simulink model "vehicle_sil"  (R2022b)
settings: Solver=VariableStepAuto  StartTime=0.0  StopTime=inf  RelTol=1e-3
undefined symbols (not defined in the file or in its folder): canChannel, MI_STATUSES
libraries: canmsglib x16, canlib x10, AMK_comms_plant_lib x1, BMS_plant_lib x1, realtime_pacer_lib x1, battery_monitor_lib x1, driver_interface_lib x1, governor_lib x1, motor_interface_lib x1, simp_vd_lib x1
settings Model: Creator=LinF  LastModifiedBy=LinF

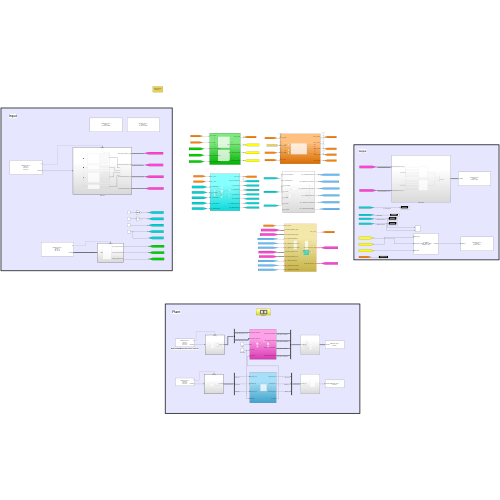
[thumbnail: Simulink's stored preview of the top-level diagram]
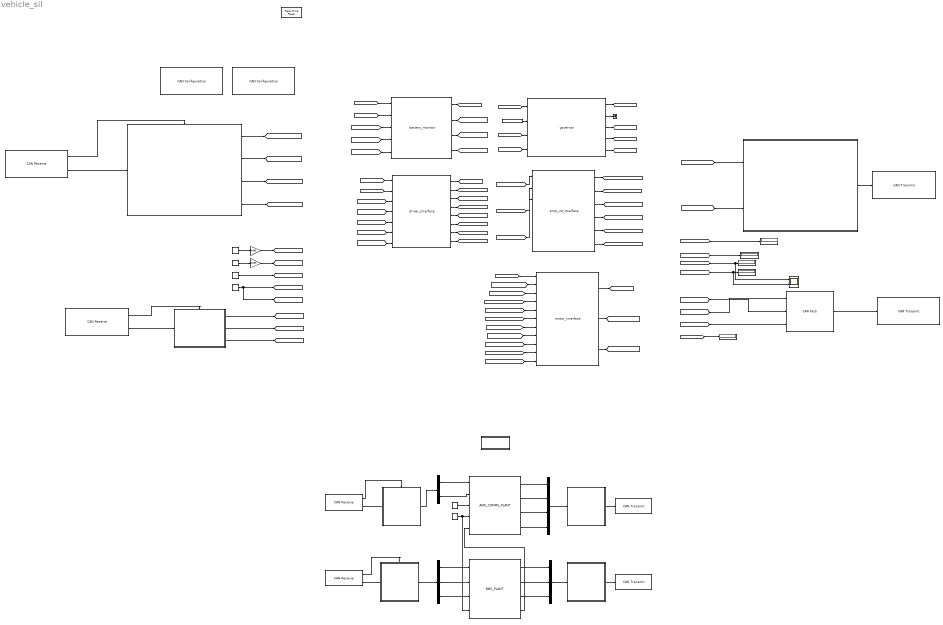
== system vehicle_sil ==
  note: Input
  note: Output
  note: Replace MathWorks with Kvaser Channels
  note: Plant
  AMK_COMMS_PLANT : AMK_comms_plant_lib/AMK_COMMS_PLANT  SystemSampleTime=-1  VariantActivationTime=update diagram  Latency=0  AutoFrameSizeCalculation=off
  AMK_Input : Subsystem  TreatAsAtomicUnit=on
  AMK_Output : Subsystem
  BMS_PLANT : BMS_plant_lib/BMS_PLANT  SystemSampleTime=-1  VariantActivationTime=update diagram  Latency=0  AutoFrameSizeCalculation=off
  Bus Creator : BusCreator  Inputs=4
  Bus Creator1 : BusCreator  Inputs=3
  Bus Selector : BusSelector  OutputSignals=ptCAN_AMK_Setpoints1_Left,ptCAN_AMK_Setpoints1_Right
  Bus Selector1 : BusSelector  OutputSignals=AIR_pos,precharge,AIR_neg
  CAN Configuration : canlib/CAN Configuration  BlockHandle=196.0002  Device=MathWorks Virtual 1 (Channel 1)  DeviceMenu=MathWorks Virtual 1 (Channel 1)  ObjConstructor=canChannel('MathWorks', 'Virtual 1', 1)  BusSpeed=500000  EnableBitParameters=off  AckMode=Normal
  CAN Configuration3 : canlib/CAN Configuration  BlockHandle=197.0002  Device=MathWorks Virtual 1 (Channel 2)  DeviceMenu=MathWorks Virtual 1 (Channel 2)  ObjConstructor=canChannel('MathWorks', 'Virtual 1', 2)  BusSpeed=500000  EnableBitParameters=off  AckMode=Normal
  CAN Pack1 : canmsglib/CAN Pack  CANdbFile=C:\Users\LinF\Documents\MACFE\Embedded\CAN_Databases\BMS.dbc  MsgList=MSGID_0X622  MsgName=MSGID_0X622  MsgIDType=Standard (11-bit identifier)  MsgIdentifier=1570  MsgLength=3  Remote=off  ApplyMinMax=off  BusOutput=off  SignalInfo={'MPO2_State','16','8','BE','unsigned','Standard','0','1','0','-Inf','Inf';'MPO4_State','8','8','BE','unsigned','Standard','0','1','0','-Inf','Inf';'MPO_State','0','8','BE','unsigned','Standard','0','1','0','-Inf','Inf'}
      settings: LibrarySourceBlock=embeddedtargetslib/Host Communication/CAN Pack  DataFormat=CANdb specified signals
  CAN Receive : canlib/CAN Receive  BlockHandle=203.0002  Device=MathWorks Virtual 1 (Channel 1)  DeviceMenu=MathWorks Virtual 1 (Channel 1)  ObjConstructor=canChannel('MathWorks', 'Virtual 1', 1)  EnableStandardIDsFilter=off  StdIDsCombo=Allow all  StandardIDs=0  EnableExtendedIDsFilter=off  ExtIDsCombo=Allow all  ExtendedIDs=0  SampleTime=0.005  MsgsPerTimestep=all  InternalFilterUpdateStatus=on  BusOutput=off
  CAN Receive1 : canlib/CAN Receive  BlockHandle=206.0002  Device=MathWorks Virtual 1 (Channel 1)  DeviceMenu=MathWorks Virtual 1 (Channel 1)  ObjConstructor=canChannel('MathWorks', 'Virtual 1', 1)  EnableStandardIDsFilter=off  StdIDsCombo=Allow all  StandardIDs=0  EnableExtendedIDsFilter=off  ExtIDsCombo=Allow all  ExtendedIDs=0  SampleTime=0.005  MsgsPerTimestep=all  InternalFilterUpdateStatus=on  BusOutput=off
  CAN Receive2 : canlib/CAN Receive  BlockHandle=209.0002  Device=MathWorks Virtual 1 (Channel 2)  DeviceMenu=MathWorks Virtual 1 (Channel 2)  ObjConstructor=canChannel('MathWorks', 'Virtual 1', 2)  EnableStandardIDsFilter=off  StdIDsCombo=Allow all  StandardIDs=0  EnableExtendedIDsFilter=off  ExtIDsCombo=Allow all  ExtendedIDs=0  SampleTime=0.005  MsgsPerTimestep=all  InternalFilterUpdateStatus=on  BusOutput=off
  CAN Receive4 : canlib/CAN Receive  BlockHandle=212.0002  Device=MathWorks Virtual 1 (Channel 2)  DeviceMenu=MathWorks Virtual 1 (Channel 2)  ObjConstructor=canChannel('MathWorks', 'Virtual 1', 2)  EnableStandardIDsFilter=off  StdIDsCombo=Allow all  StandardIDs=0  EnableExtendedIDsFilter=off  ExtIDsCombo=Allow all  ExtendedIDs=0  SampleTime=0.005  MsgsPerTimestep=all  InternalFilterUpdateStatus=on  BusOutput=on
  CAN Transmit : canlib/CAN Transmit  BlockHandle=215.0002  Device=MathWorks Virtual 1 (Channel 1)  DeviceMenu=MathWorks Virtual 1 (Channel 1)  ObjConstructor=canChannel('MathWorks', 'Virtual 1', 1)  EnableEventTransmit=off  EnablePeriodicTransmit=on  MessagePeriod=0.005
  CAN Transmit1 : canlib/CAN Transmit  BlockHandle=217.0002  Device=MathWorks Virtual 1 (Channel 1)  DeviceMenu=MathWorks Virtual 1 (Channel 1)  ObjConstructor=canChannel('MathWorks', 'Virtual 1', 1)  EnableEventTransmit=off  EnablePeriodicTransmit=off  MessagePeriod=1.000
  CAN Transmit2 : canlib/CAN Transmit  BlockHandle=219.0002  Device=MathWorks Virtual 1 (Channel 2)  DeviceMenu=MathWorks Virtual 1 (Channel 2)  ObjConstructor=canChannel('MathWorks', 'Virtual 1', 2)  EnableEventTransmit=off  EnablePeriodicTransmit=off  MessagePeriod=1.000
  CAN Transmit4 : canlib/CAN Transmit  BlockHandle=221.0002  Device=MathWorks Virtual 1 (Channel 2)  DeviceMenu=MathWorks Virtual 1 (Channel 2)  ObjConstructor=canChannel('MathWorks', 'Virtual 1', 2)  EnableEventTransmit=off  EnablePeriodicTransmit=on  MessagePeriod=0.005
  Constant : Constant  Value=MI_STATUSES.STS_INIT  OutDataTypeStr=Enum: MI_STATUSES
  Constant1 : Constant  VectorParams1D=off
  Constant4 : Constant  Value=0
  Constant5 : Constant  Value=0
  Constant7 : Constant  Value=0
  Dashboard : Subsystem
  Display{,1..4} (5 alike) : Display
  Function-Call Subsystem : Subsystem  TreatAsAtomicUnit=on
  Function-Call Subsystem1 : Subsystem  TreatAsAtomicUnit=on
  Function-Call Subsystem2 : Subsystem  TreatAsAtomicUnit=on
  Gain : Gain  Gain=4095
  Gain1 : Gain  Gain=4095
  LV_Enable : Constant
  Real-Time Pacer : realtime_pacer_lib/Real-Time Pacer  simTimePerRealTime=1
  Scope1 : Scope  NumInputPorts=2
  Subsystem : Subsystem
  Subsystem1 : Subsystem
  Terminator : Terminator
  X140 : Constant
  battery_monitor : battery_monitor_lib/battery_monitor  SystemSampleTime=-1  VariantActivationTime=update diagram  Latency=0  AutoFrameSizeCalculation=off
  driver_interface : driver_interface_lib/driver_interface  SystemSampleTime=-1  VariantActivationTime=update diagram  Latency=0  AutoFrameSizeCalculation=off
  governor : governor_lib/governor  SystemSampleTime=-1  VariantActivationTime=update diagram  Latency=0  AutoFrameSizeCalculation=off
  motor_interface : motor_interface_lib/motor_interface  SystemSampleTime=-1  VariantActivationTime=update diagram  Latency=0  AutoFrameSizeCalculation=off
  simp_vd_interface : simp_vd_lib/simp_vd_interface  SystemSampleTime=-1  VariantActivationTime=update diagram  Latency=0  AutoFrameSizeCalculation=off
  wires:
  Constant7/1 -> [DI_V_AccelPedalPos2], [DI_V_AccelPedalPos1]
  [DI_b_driverSpeaker] -> Display/1  "DI_b_driverSpeaker"
  Constant4/1 -> Gain/1
  Gain1/1 -> [DI_V_BrakePedalPos]
  motor_interface/1 -> [GOV_e_miSts]
  [ptCAN_AMK_Setpoints1_Right] -> AMK_Output/1(ptCAN_AMK_Setpoints1_Right)  "ptCAN_AMK_Setpoints1_Right"
  Constant5/1 -> Gain1/1
  [VD_T_RightMotorTorqueLimitPositive] -> motor_interface/5
  AMK_Input/2(ptCAN_AMK_ActualValues2_Right) -> [ptCAN_AMK_ActualValues2_Right]
  CAN Receive/1 -> AMK_Input/Trigger
  AMK_Output/1(Out1) -> CAN Transmit/1
  AMK_Input/4(ptCAN_AMK_ActualValues2_Left) -> [ptCAN_AMK_ActualValues2_Left]
  AMK_Input/3(ptCAN_AMK_ActualValues1_Left) -> [ptCAN_AMK_ActualValues1_Left]
  CAN Receive/2 -> AMK_Input/1(In1)
  motor_interface/3 -> [ptCAN_AMK_Setpoints1_Left]
  motor_interface/2 -> [ptCAN_AMK_Setpoints1_Right]
  [VD_T_LeftMotorTorqueLimitPositive] -> motor_interface/10
  [VD_T_RightMotorTorqueLimitNegative] -> motor_interface/6
  [VD_n_RightMotorSpeedRequest] -> motor_interface/4
  [GOV_e_miCmd] -> motor_interface/1
  [VD_T_LeftMotorTorqueLimitNegative] -> motor_interface/11
  [VD_n_LeftMotorSpeedRequest] -> motor_interface/9
  AMK_Input/1(ptCAN_AMK_ActualValues1_Right) -> [ptCAN_AMK_ActualValues1_Right]
  [ptCAN_AMK_ActualValues2_Left] -> motor_interface/8
  [ptCAN_AMK_ActualValues1_Right] -> motor_interface/2
  [ptCAN_AMK_ActualValues2_Right] -> motor_interface/3
  [ptCAN_AMK_ActualValues1_Left] -> motor_interface/7
  [ptCAN_AMK_Setpoints1_Left] -> AMK_Output/2(ptCAN_AMK_Setpoints1_Left)  "ptCAN_AMK_Setpoints1_Left"
  Gain/1 -> [DI_V_SteeringAngle]
  [BM_b_HVnegContactorSts] -> battery_monitor/5
  [GOV_e_bmCmd] -> battery_monitor/1
  battery_monitor/1 -> [GOV_e_bmSts]
  battery_monitor/2 -> [BM_b_prechargeContactorCMD]
  battery_monitor/3 -> [BM_b_HVposContactorCMD]
  [BM_b_prechrgContactorSts] -> battery_monitor/3
  battery_monitor/4 -> [BM_b_HVnegContactorCMD]
  [BM_b_HVposContactorSts] -> battery_monitor/4
  [GOV_e_diSts] -> battery_monitor/2
  [DI_b_brakeLightEn] -> Display4/1  "DI_b_brakeLightEn"
  [DI_p_PWMstatusLightFreq] -> Scope1/2, Display2/1  "DI_p_PWMstatusLightFreq"
  [DI_p_PWMstatusLightCycle] -> Scope1/1, Display1/1  "DI_p_PWMstatusLightCycle"
  simp_vd_interface/4 -> [VD_n_LeftMotorSpeedRequest]
  simp_vd_interface/2 -> [VD_T_RightMotorTorqueLimitPositive]
  [DI_p_driverTorqueRequest] -> simp_vd_interface/1
  simp_vd_interface/6 -> [VD_T_LeftMotorTorqueLimitNegative]
  simp_vd_interface/3 -> [VD_T_RightMotorTorqueLimitNegative]
  [DI_p_steeringAngle] -> simp_vd_interface/3
  [DI_p_brakePedalPosition] -> simp_vd_interface/2
  simp_vd_interface/5 -> [VD_T_LeftMotorTorqueLimitPositive]
  simp_vd_interface/1 -> [VD_n_RightMotorSpeedRequest]
  BMS_PLANT/4 -> AMK_COMMS_PLANT/5
  AMK_COMMS_PLANT/4 -> Bus Creator/4  "ptCAN_AMK1_ActualValues2"
  AMK_COMMS_PLANT/3 -> Bus Creator/3  "ptCAN_AMK1_ActualValues1"
  Bus Creator/1 -> Subsystem/1(pt_CAN_OUT)
  CAN Receive1/1 -> Function-Call Subsystem/Trigger
  BMS_PLANT/2 -> Bus Creator1/2  "precharge_sts"
  Subsystem/1(Out1) -> CAN Transmit1/1
  Bus Selector1/2 -> BMS_PLANT/2  "<precharge>"
  Function-Call Subsystem1/1(pt_CAN_IN) -> Bus Selector1/1
  BMS_PLANT/3 -> Bus Creator1/3  "AIR_neg_sts"
  CAN Receive2/1 -> Function-Call Subsystem1/Trigger
  AMK_COMMS_PLANT/2 -> Bus Creator/2  "ptCAN_AMK0_ActualValues2"
  Function-Call Subsystem/1(pt_CAN_IN) -> Bus Selector/1
  Bus Selector1/1 -> BMS_PLANT/1  "<AIR_pos>"
  CAN Receive2/2 -> Function-Call Subsystem1/1(In1)
  AMK_COMMS_PLANT/1 -> Bus Creator/1  "ptCAN_AMK0_ActualValues1"
  BMS_PLANT/1 -> Bus Creator1/1  "AIR_pos_sts"
  Bus Selector/2 -> AMK_COMMS_PLANT/2  "<ptCAN_AMK_Setpoints1_Right>"
  X140/1 -> AMK_COMMS_PLANT/3
  Bus Selector1/3 -> BMS_PLANT/3  "<AIR_neg>"
  LV_Enable/1 -> BMS_PLANT/4, AMK_COMMS_PLANT/4
  Subsystem1/1(Out1) -> CAN Transmit2/1
  Bus Selector/1 -> AMK_COMMS_PLANT/1  "<ptCAN_AMK_Setpoints1_Left>"
  CAN Receive1/2 -> Function-Call Subsystem/1(In1)
  Bus Creator1/1 -> Subsystem1/1(pt_CAN_OUT)
  CAN Receive4/1 -> Function-Call Subsystem2/Trigger
  Function-Call Subsystem2/1(BM_b_prechrgContactorSts) -> [BM_b_prechrgContactorSts]
  CAN Receive4/2 -> Function-Call Subsystem2/1(In1)
  Function-Call Subsystem2/2(BM_b_HVposContactorSts) -> [BM_b_HVposContactorSts]
  Function-Call Subsystem2/3(BM_b_HVnegContactorSts) -> [BM_b_HVnegContactorSts]
  CAN Pack1/1 -> CAN Transmit4/1
  [BM_b_prechargeContactorCMD] -> CAN Pack1/2
  [BM_b_HVposContactorCMD] -> CAN Pack1/1
  [BM_b_HVnegContactorCMD] -> CAN Pack1/3
  driver_interface/5 -> [DI_b_driverSpeaker]
  [GOV_e_miSts] -> driver_interface/1
  [GOV_e_diCmd] -> driver_interface/2
  driver_interface/4 -> [DI_p_brakePedalPosition]
  [DI_V_AccelPedalPos2] -> driver_interface/6
  [DI_V_SteeringAngle] -> driver_interface/7
  driver_interface/2 -> [DI_p_driverTorqueRequest]
  driver_interface/1 -> [GOV_e_diSts]
  [DI_V_BrakePedalPos] -> driver_interface/3
  driver_interface/7 -> [DI_p_PWMstatusLightCycle]
  [DI_V_AccelPedalPos1] -> driver_interface/5
  driver_interface/6 -> [DI_b_brakeLightEn]
  driver_interface/3 -> [DI_p_steeringAngle]
  driver_interface/8 -> [DI_p_PWMstatusLightFreq]
  [DI_b_DriverButton] -> driver_interface/4
  governor/5 -> [GOV_e_govSts]
  [GOV_e_diSts] -> governor/4
  [GOV_e_bmSts] -> governor/1
  [GOV_e_miSts] -> governor/3
  governor/3 -> [GOV_e_miCmd]
  governor/1 -> [GOV_e_bmCmd]
  governor/4 -> [GOV_e_diCmd]
  governor/2 -> Terminator/1
  Constant/1 -> governor/2
  [GOV_e_govSts] -> Display3/1
  Constant1/1 -> [DI_b_DriverButton]

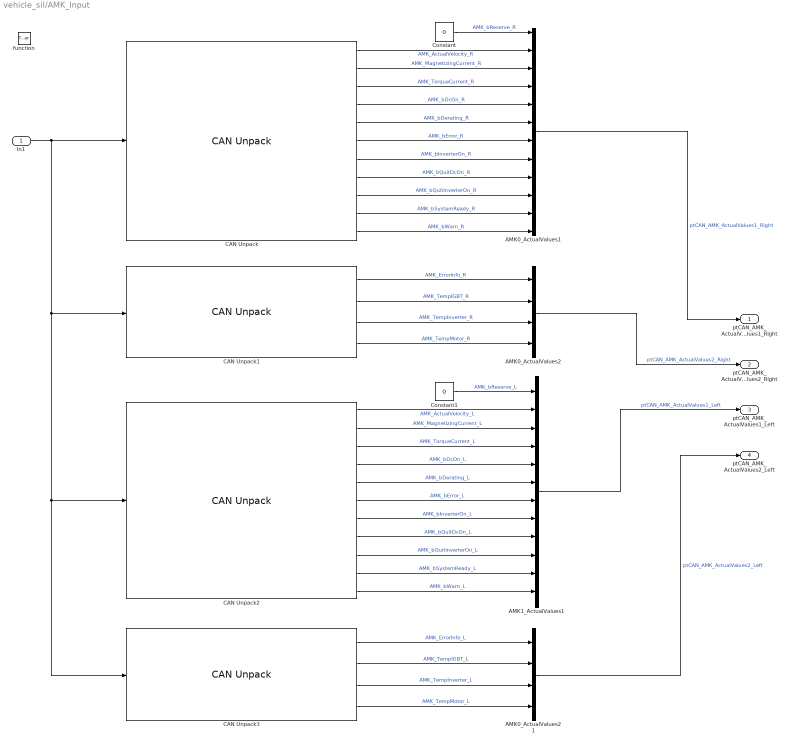
== system vehicle_sil/AMK_Input ==
  In1 : Inport
  function : TriggerPort  TriggerType=function-call  VariantControl=(inherit)
  "AMK0_ActualValues1 " : BusCreator  Inputs=12
  "AMK0_ActualValues2 " : BusCreator  Inputs=4
  AMK0_ActualValues2 1 : BusCreator  Inputs=4
  AMK1_ActualValues1 : BusCreator  Inputs=12
  CAN Unpack : canmsglib/CAN Unpack  CANdbFile=C:\Users\LinF\Documents\MACFE\Embedded\CAN_Stuff\CAN_Databases\CAN_AMKInverter.dbc  MsgList=AMK1_ActualValues1  MsgName=AMK1_ActualValues1  MsgIDType=Standard (11-bit identifier)  MsgIdentifier=645  MsgLength=8  SignalInfo={'AMK_ActualVelocity','16','16','LE','signed','Standard','0','1','0','-Inf','Inf';'AMK_MagnetizingCurrent','48','16','LE','signed','Standard','0','1','0','-Inf','Inf';'AMK_TorqueCurrent','32','16','LE','signed','Standard','0','1','0','-Inf','Inf';'AMK_bDcOn','12','1','LE','unsigned','Standard','0','1','0','-Inf','Inf';'AMK_bDerating','15','1','LE','unsigned','Standard','0','1','0','-Inf','Inf';'AMK_bError','9','1','LE','unsigned','Standard','0','1','0','-Inf','Inf';'AMK_bInverterOn','14','1','LE','unsigned','Standard','0','1','0','-Inf','Inf';'AMK_bQuitDcOn','11','1','LE','unsigned','Standard','0','1','0','-Inf','Inf';'AMK_bQuitInverterOn','13','1','LE','unsigned','Standard','0','1','0','-Inf','Inf';'AMK_bSystemReady','8','1','LE','unsigned','Standard','0','1','0','-Inf','Inf';'AMK_bWarn','10','1','LE','unsigned','Standard','0','1','0','-Inf','Inf'}  IDPort=off  TimestampPort=off  ErrorPort=off  RemotePort=off  LengthPort=off  StatusPort=off  ApplyMinMax=off
      settings: LibrarySourceBlock=canlib/CAN Unpack  DataFormat=CANdb specified signals
  CAN Unpack1 : canmsglib/CAN Unpack  CANdbFile=C:\Users\LinF\Documents\MACFE\Embedded\CAN_Stuff\CAN_Databases\CAN_AMKInverter.dbc  MsgList=AMK1_ActualValues2  MsgName=AMK1_ActualValues2  MsgIDType=Standard (11-bit identifier)  MsgIdentifier=647  MsgLength=8  SignalInfo={'AMK_ErrorInfo','32','16','LE','unsigned','Standard','0','1','0','0','65535';'AMK_TempIGBT','48','16','LE','signed','Standard','0','0.1','0','-3276.8','3276.7';'AMK_TempInverter','16','16','LE','signed','Standard','0','0.1','0','-3276.8','3276.7';'AMK_TempMotor','0','16','LE','signed','Standard','0','0.1','0','-3276.8','3276.7'}  IDPort=off  TimestampPort=off  ErrorPort=off  RemotePort=off  LengthPort=off  StatusPort=off  ApplyMinMax=off
      settings: LibrarySourceBlock=canlib/CAN Unpack  DataFormat=CANdb specified signals
  CAN Unpack2 : canmsglib/CAN Unpack  CANdbFile=C:\Users\LinF\Documents\MACFE\Embedded\CAN_Stuff\CAN_Databases\CAN_AMKInverter.dbc  MsgList=AMK0_ActualValues1  MsgName=AMK0_ActualValues1  MsgIDType=Standard (11-bit identifier)  MsgIdentifier=644  MsgLength=8  SignalInfo={'AMK_ActualVelocity','16','16','LE','signed','Standard','0','1','0','-Inf','Inf';'AMK_MagnetizingCurrent','48','16','LE','signed','Standard','0','1','0','-Inf','Inf';'AMK_TorqueCurrent','32','16','LE','signed','Standard','0','1','0','-Inf','Inf';'AMK_bDcOn','12','1','LE','unsigned','Standard','0','1','0','-Inf','Inf';'AMK_bDerating','15','1','LE','unsigned','Standard','0','1','0','-Inf','Inf';'AMK_bError','9','1','LE','unsigned','Standard','0','1','0','-Inf','Inf';'AMK_bInverterOn','14','1','LE','unsigned','Standard','0','1','0','-Inf','Inf';'AMK_bQuitDcOn','11','1','LE','unsigned','Standard','0','1','0','-Inf','Inf';'AMK_bQuitInverterOn','13','1','LE','unsigned','Standard','0','1','0','-Inf','Inf';'AMK_bSystemReady','8','1','LE','unsigned','Standard','0','1','0','-Inf','Inf';'AMK_bWarn','10','1','LE','unsigned','Standard','0','1','0','-Inf','Inf'}  IDPort=off  TimestampPort=off  ErrorPort=off  RemotePort=off  LengthPort=off  StatusPort=off  ApplyMinMax=off
      settings: LibrarySourceBlock=canlib/CAN Unpack  DataFormat=CANdb specified signals
  CAN Unpack3 : canmsglib/CAN Unpack  CANdbFile=C:\Users\LinF\Documents\MACFE\Embedded\CAN_Stuff\CAN_Databases\CAN_AMKInverter.dbc  MsgList=AMK0_ActualValues2  MsgName=AMK0_ActualValues2  MsgIDType=Standard (11-bit identifier)  MsgIdentifier=646  MsgLength=8  SignalInfo={'AMK_ErrorInfo','32','16','LE','unsigned','Standard','0','1','0','0','65535';'AMK_TempIGBT','48','16','LE','signed','Standard','0','0.1','0','-3276.8','3276.7';'AMK_TempInverter','16','16','LE','signed','Standard','0','0.1','0','-3276.8','3276.7';'AMK_TempMotor','0','16','LE','signed','Standard','0','0.1','0','-3276.8','3276.7'}  IDPort=off  TimestampPort=off  ErrorPort=off  RemotePort=off  LengthPort=off  StatusPort=off  ApplyMinMax=off
      settings: LibrarySourceBlock=canlib/CAN Unpack  DataFormat=CANdb specified signals
  Constant : Constant  Value=0
  Constant1 : Constant  Value=0
  ptCAN_AMK_ActualValues1_Right : Outport
  ptCAN_AMK_ActualValues2_Right : Outport  Port=2
  ptCAN_AMK_ActualValues1_Left : Outport  Port=3
  ptCAN_AMK_ActualValues2_Left : Outport  Port=4
  wires:
  In1/1 -> CAN Unpack3/1, CAN Unpack2/1, CAN Unpack1/1, CAN Unpack/1
  CAN Unpack/1 -> "AMK0_ActualValues1 "/2  "AMK_ActualVelocity_R"
  CAN Unpack/2 -> "AMK0_ActualValues1 "/3  "AMK_MagnetizingCurrent_R"
  CAN Unpack/3 -> "AMK0_ActualValues1 "/4  "AMK_TorqueCurrent_R"
  CAN Unpack/4 -> "AMK0_ActualValues1 "/5  "AMK_bDcOn_R"
  CAN Unpack/5 -> "AMK0_ActualValues1 "/6  "AMK_bDerating_R"
  CAN Unpack/6 -> "AMK0_ActualValues1 "/7  "AMK_bError_R"
  CAN Unpack/7 -> "AMK0_ActualValues1 "/8  "AMK_bInverterOn_R"
  CAN Unpack/8 -> "AMK0_ActualValues1 "/9  "AMK_bQuitDcOn_R"
  CAN Unpack/9 -> "AMK0_ActualValues1 "/10  "AMK_bQuitInverterOn_R"
  CAN Unpack/10 -> "AMK0_ActualValues1 "/11  "AMK_bSystemReady_R"
  CAN Unpack/11 -> "AMK0_ActualValues1 "/12  "AMK_bWarn_R"
  "AMK0_ActualValues1 "/1 -> ptCAN_AMK_ActualValues1_Right/1  "ptCAN_AMK_ActualValues1_Right"
  CAN Unpack2/1 -> AMK1_ActualValues1/2  "AMK_ActualVelocity_L"
  CAN Unpack2/10 -> AMK1_ActualValues1/11  "AMK_bSystemReady_L"
  CAN Unpack2/6 -> AMK1_ActualValues1/7  "AMK_bError_L"
  CAN Unpack2/9 -> AMK1_ActualValues1/10  "AMK_bQuitInverterOn_L"
  CAN Unpack2/2 -> AMK1_ActualValues1/3  "AMK_MagnetizingCurrent_L"
  CAN Unpack2/3 -> AMK1_ActualValues1/4  "AMK_TorqueCurrent_L"
  AMK1_ActualValues1/1 -> ptCAN_AMK_ActualValues1_Left/1  "ptCAN_AMK_ActualValues1_Left"
  CAN Unpack2/8 -> AMK1_ActualValues1/9  "AMK_bQuitDcOn_L"
  CAN Unpack2/4 -> AMK1_ActualValues1/5  "AMK_bDcOn_L"
  CAN Unpack2/5 -> AMK1_ActualValues1/6  "AMK_bDerating_L"
  CAN Unpack2/11 -> AMK1_ActualValues1/12  "AMK_bWarn_L"
  CAN Unpack2/7 -> AMK1_ActualValues1/8  "AMK_bInverterOn_L"
  CAN Unpack1/1 -> "AMK0_ActualValues2 "/1  "AMK_ErrorInfo_R"
  CAN Unpack1/2 -> "AMK0_ActualValues2 "/2  "AMK_TempIGBT_R"
  CAN Unpack1/3 -> "AMK0_ActualValues2 "/3  "AMK_TempInverter_R"
  CAN Unpack1/4 -> "AMK0_ActualValues2 "/4  "AMK_TempMotor_R"
  "AMK0_ActualValues2 "/1 -> ptCAN_AMK_ActualValues2_Right/1  "ptCAN_AMK_ActualValues2_Right"
  CAN Unpack3/1 -> AMK0_ActualValues2 1/1  "AMK_ErrorInfo_L"
  CAN Unpack3/4 -> AMK0_ActualValues2 1/4  "AMK_TempMotor_L"
  AMK0_ActualValues2 1/1 -> ptCAN_AMK_ActualValues2_Left/1  "ptCAN_AMK_ActualValues2_Left"
  CAN Unpack3/3 -> AMK0_ActualValues2 1/3  "AMK_TempInverter_L"
  CAN Unpack3/2 -> AMK0_ActualValues2 1/2  "AMK_TempIGBT_L"
  Constant/1 -> "AMK0_ActualValues1 "/1  "AMK_bReserve_R"
  Constant1/1 -> AMK1_ActualValues1/1  "AMK_bReserve_L"

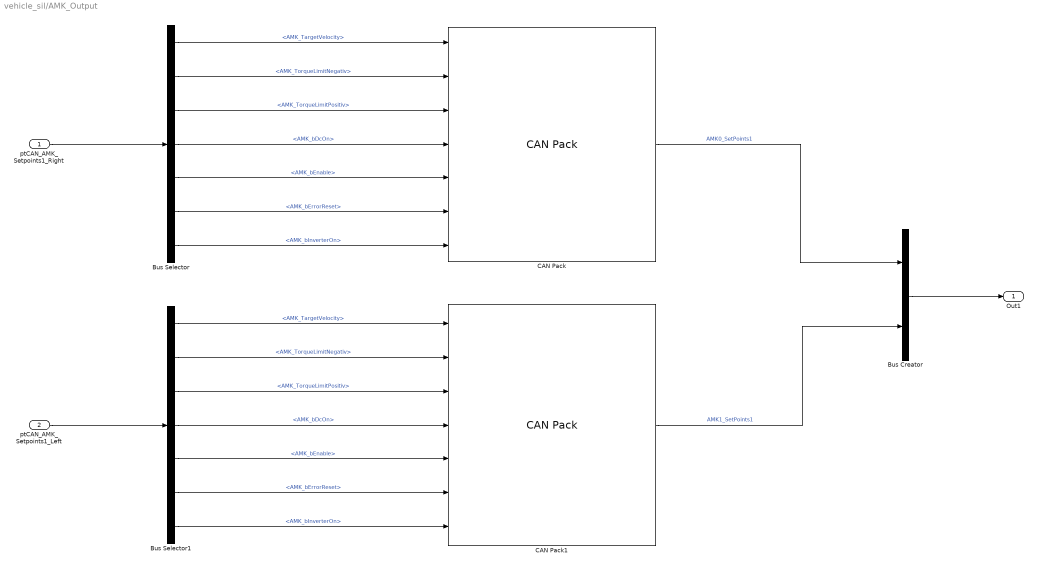
== system vehicle_sil/AMK_Output ==
  ptCAN_AMK_Setpoints1_Right : Inport
  ptCAN_AMK_Setpoints1_Left : Inport  Port=2
  Bus Creator : BusCreator  Inputs=2
  Bus Selector : BusSelector  OutputSignals=AMK_TargetVelocity,AMK_TorqueLimitNegativ,AMK_TorqueLimitPositiv,AMK_bDcOn,AMK_bEnable,AMK_bErrorReset,AMK_bInverterOn
  Bus Selector1 : BusSelector  OutputSignals=AMK_TargetVelocity,AMK_TorqueLimitNegativ,AMK_TorqueLimitPositiv,AMK_bDcOn,AMK_bEnable,AMK_bErrorReset,AMK_bInverterOn
  CAN Pack : canmsglib/CAN Pack  CANdbFile=C:\Users\LinF\Documents\MACFE\Embedded\CAN_Stuff\CAN_Databases\CAN_AMKInverter.dbc  MsgList=AMK1_SetPoints1  MsgName=AMK1_SetPoints1  MsgIDType=Standard (11-bit identifier)  MsgIdentifier=390  MsgLength=8  Remote=off  ApplyMinMax=off  BusOutput=off  SignalInfo={'AMK_TargetVelocity','16','16','LE','signed','Standard','0','1','0','-Inf','Inf';'AMK_TorqueLimitNegativ','48','16','LE','signed','Standard','0','1','0','-Inf','Inf';'AMK_TorqueLimitPositiv','32','16','LE','signed','Standard','0','1','0','-Inf','Inf';'AMK_bDcOn','9','1','LE','unsigned','Standard','0','1','0','-Inf','Inf';'AMK_bEnable','10','1','LE','unsigned','Standard','0','1','0','-Inf','Inf';'AMK_bErrorReset','11','1','LE','unsigned','Standard','0','1','0','-Inf','Inf';'AMK_bInverterOn','8','1','LE','unsigned','Standard','0','1','0','-Inf','Inf'}
      settings: LibrarySourceBlock=canlib/CAN Pack  DataFormat=CANdb specified signals
  CAN Pack1 : canmsglib/CAN Pack  CANdbFile=C:\Users\LinF\Documents\MACFE\Embedded\CAN_Stuff\CAN_Databases\CAN_AMKInverter.dbc  MsgList=AMK0_SetPoints1  MsgName=AMK0_SetPoints1  MsgIDType=Standard (11-bit identifier)  MsgIdentifier=389  MsgLength=8  Remote=off  ApplyMinMax=off  BusOutput=off  SignalInfo={'AMK_TargetVelocity','16','16','LE','signed','Standard','0','1','0','-Inf','Inf';'AMK_TorqueLimitNegativ','48','16','LE','signed','Standard','0','1','0','-Inf','Inf';'AMK_TorqueLimitPositiv','32','16','LE','signed','Standard','0','1','0','-Inf','Inf';'AMK_bDcOn','9','1','LE','unsigned','Standard','0','1','0','-Inf','Inf';'AMK_bEnable','10','1','LE','unsigned','Standard','0','1','0','-Inf','Inf';'AMK_bErrorReset','11','1','LE','unsigned','Standard','0','1','0','-Inf','Inf';'AMK_bInverterOn','8','1','LE','unsigned','Standard','0','1','0','-Inf','Inf'}
      settings: LibrarySourceBlock=canlib/CAN Pack  DataFormat=CANdb specified signals
  Out1 : Outport
  wires:
  CAN Pack/1 -> Bus Creator/1  "AMK0_SetPoints1"
  CAN Pack1/1 -> Bus Creator/2  "AMK1_SetPoints1"
  Bus Selector/7 -> CAN Pack/7  "<AMK_bInverterOn>"
  Bus Selector/4 -> CAN Pack/4  "<AMK_bDcOn>"
  Bus Selector/5 -> CAN Pack/5  "<AMK_bEnable>"
  Bus Selector/6 -> CAN Pack/6  "<AMK_bErrorReset>"
  Bus Selector/1 -> CAN Pack/1  "<AMK_TargetVelocity>"
  Bus Selector/3 -> CAN Pack/3  "<AMK_TorqueLimitPositiv>"
  Bus Selector/2 -> CAN Pack/2  "<AMK_TorqueLimitNegativ>"
  Bus Creator/1 -> Out1/1
  Bus Selector1/1 -> CAN Pack1/1  "<AMK_TargetVelocity>"
  Bus Selector1/3 -> CAN Pack1/3  "<AMK_TorqueLimitPositiv>"
  Bus Selector1/2 -> CAN Pack1/2  "<AMK_TorqueLimitNegativ>"
  Bus Selector1/4 -> CAN Pack1/4  "<AMK_bDcOn>"
  Bus Selector1/5 -> CAN Pack1/5  "<AMK_bEnable>"
  Bus Selector1/6 -> CAN Pack1/6  "<AMK_bErrorReset>"
  Bus Selector1/7 -> CAN Pack1/7  "<AMK_bInverterOn>"
  ptCAN_AMK_Setpoints1_Right/1 -> Bus Selector/1
  ptCAN_AMK_Setpoints1_Left/1 -> Bus Selector1/1

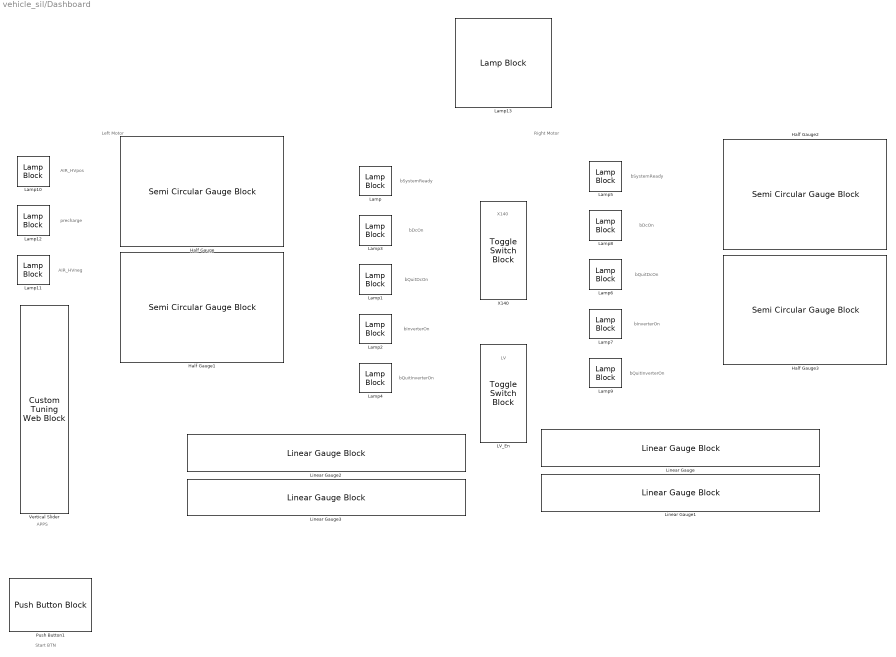
== system vehicle_sil/Dashboard ==
  note: Start BTN
  note: APPS
  note: LV
  note: X140
  note: Left Motor
  note: bQuitInverterOn
  note: bInverterOn
  note: bQuitDcOn
  note: bDcOn
  note: bSystemReady
  note: bDcOn
  note: bQuitDcOn
  note: bSystemReady
  note: bInverterOn
  note: bQuitInverterOn
  note: Right Motor
  note: AIR_HVpos
  note: precharge
  note: AIR_HVneg
  Half Gauge : SemiCircularGaugeBlock  LabelPosition=Bottom  ScaleMax=20000  TickInterval=2000
  Half Gauge1 : SemiCircularGaugeBlock  LabelPosition=Bottom  ScaleMax=1000  TickInterval=100
  Half Gauge2 : SemiCircularGaugeBlock  LabelPosition=Bottom  ScaleMax=20000  TickInterval=2000
  Half Gauge3 : SemiCircularGaugeBlock  LabelPosition=Bottom  ScaleMax=1000  TickInterval=100
  LV_En : ToggleSwitchBlock  LabelPosition=Bottom
      settings: Values={{'Off', 'On'}, [0 1]}
  Lamp{,1..13} (14 alike) : LampBlock  LabelPosition=Hide
  Linear Gauge : LinearGaugeBlock  ScaleMax=20000  TickInterval=2000
  Linear Gauge1 : LinearGaugeBlock  ScaleMax=1000  TickInterval=100
  Linear Gauge2 : LinearGaugeBlock  ScaleMax=20000  TickInterval=2000
  Linear Gauge3 : LinearGaugeBlock  ScaleMax=1000  TickInterval=100
  Push Button1 : PushButtonBlock  OnValue=0  OffValue=1.000000
  Vertical Slider : CustomTuningWebBlock  LabelPosition=Hide  ShowInitialText=on  Configuration="{\"components\":[{\"name\":\"LinearScaleComponent\",\"settings\":{\"bounds\":{\"max\":5000,\"min\":0,\"tickInterval\":\"auto\"},\"internalTickHeightScaleFactor\":0.5,\"labelColor\":[255,255,200],\"labelFont\":{\"font\":\"Arial\",\"fontSize\":12},\"labelOffset\":0.05,\"labelTransparency\":1,\"needleImage\":{\"size\":[596,842],\"src\":\"data:image\\/svg+xml;base64,PD94bWwgdmVyc2lvbj0iMS4wIiBlbmNvZGluZz0idXRmLTgiPz4NCjwhLS0gR2VuZXJhdG9yOiBBZG9iZSBJbGx1c3RyYXRvciAyNS4wLjAsIFNWRyBFeHBvcnQgUGx1Zy1JbiAuIFNWRyBWZXJzaW9uOiA2LjAwIEJ1aWxkIDApICAtLT4NCjxzdmcgdmVyc2lvbj0iMS4xIg0KCSBpZD0ic3ZnOCIgeG1sbnM6Y2M9Imh0dHA6Ly9jcmVhdGl2ZWNvbW1vbnMub3JnL25zIyIgeG1sbnM6ZGM9Imh0dHA6Ly9wdXJsLm9yZy9kYy9lbGVtZW50cy8xLjEvIiB4bWxuczppbmtzY2FwZT0iaHR0cDovL3d3dy5pbmtzY2FwZS5vcmcvbmFtZXNw ...(+2420 chars)\",\"srcOrientation\":\"horizontal\"},\"needleOffset\":[0.0642123287671233,-0.8044596912521441],\"needleSize\":{\"height\":0.07668067226890757,\"width\":0.4337797619047619},\"position\":[0.03623949579831933,0.2829861111111111,0.6088789682539683,0.9196428571428571],\"referencePoint\":\"auto\",\"scaleColors\":[],\"scaleColorsSize\":0.2,\"scaleDirection\":\"BT\",\"showLabels\":1,\"showMinorTicks\":0,\"showSpanLine\":1,\"showTicks\":1,\"tickColor\":[252,252,197],\"tickTransparency\":1,\"valueBarColor\":[0,114,189],\"valueBarOffset\":-0.27,\"valueBarSize\":0.1,\"valueBarTransparency\":1}},{\"name\":\"BackgroundImageComponent\",\"settings\":{\"image\":{\"size\":[380,101],\"src\":\"data:image\\/svg+xml;base64,PHN2ZyB4bWxucz0iaHR0cDovL3d3dy53My5vcmcvMjAwMC9zdmciIHhtbG5zOnhsaW5rPSJodHRwOi8vd3d3LnczLm9yZy8xOTk5L3hsaW5rIiB2aWV3Qm94PSIwIDAgMzgwIDEwMSI+PGRlZnM+PHN0eWxlPi5jbHMtMXtmaWxsOiMwMDJiNDI7fS5jbHMtMntmaWxsOiM0MjcwODI7fS5jbHMtM3tmaWxsOnVybCgjcmFkaWFsLWdyYWRpZW50KTt9LmNscy00e2ZpbGw6I2M4YzhjODtzdHJva2U6IzAwMDt9PC9zdHlsZT48cmFkaWFsR3JhZGllbnQgaWQ9InJhZGlhbC1ncmFkaWVudCIgY3g9IjE5MCIgY3k9IjUwLjUiIHI9IjI2OS4yMSIgZ3JhZGllbnRVbml0cz0idXNlclNwYWNlT25Vc2UiPjxzdG9wIG9mZnNldD0iMC4wMSIgc3RvcC1jb2xvcj0iIzNlNGY1OCIvPjxzdG9wIG9mZnNldD0iMC4wNiIgc3RvcC1jb2xvcj0iIzQ0NTc2MSIvPjxzdG9wIG9mZnNldD0iMC4xNSIgc3RvcC1jb2xvcj0iIzU1NmE3NiIvPjxzdG9wIG9mZnNldD0iMC4yNSIgc3RvcC1jb2xvcj0iIzZkODg5NSIvPjxzdG9wIG9mZnNldD0iMC4zOCIgc3RvcC1jb2xvcj0iIzhmYjJjMyIvPjxzdG9wIG9mZnNldD0iMC41MiIgc3RvcC1jb2xvcj0iI2I2ZTRmYSIvPjxzdG9wIG9mZnNldD0iMSIgc3RvcC1jb2xvcj0iIzE1NDY1NyIvPjwvcmFkaWFsR3JhZGllbnQ+PC9kZWZzPjxnIGlkPSJmcmFtZSI+PGcgaWQ9IkxheWVyXzIiIGRhdGEtbmFtZT0iTGF5ZXIgMiI+PGcgaWQ9IkxheWVyXzEtMiIgZGF0YS1uYW1lPSJMYXllciAxLTIiPjxyZWN0IGlkPSJyZWN0MTAzNiIgY2xhc3M9ImNscy0xIiB4PSIxMSIgeT0iMTEiIHdpZHRoPSIzNTgiIGhlaWdodD0iNzkiLz48cGF0aCBpZD0icGF0aDEwMzgiIGNsYXNzPSJjbHMtMiIgZD0iTTgsOFY5M0gzNzJWOFpNMzY5LDkwSDExVjExSDM2OVoiLz48cGF0aCBpZD0icGF0aDEwNDAiIGNsYXNzPSJjbHMtMyIgZD0iTTAsMFYxMDFIMzgwVjBaTTM3Miw5M0g4VjhIMzcyWiIvPjwvZz48L2c+PC9nPjxnIGlkPSJ0cmFjayI+PHBhdGggaWQ9InJlY3QxNjExIiBjbGFzcz0iY2xzLTQiIGQ9Ik0zMy4zNywyNi41OUgzNDYuNjNjNCwwLDcuMjUsMi42LDcuMjUsNS44MWgwYzAsMy4yMS0zLjI1LDUuODItNy4yNSw1LjgySDMzLjM3Yy00LDAtNy4yNS0yLjYxLTcuMjUtNS44MmgwQzI2LjEyLDI5LjE5LDI5LjM3LDI2LjU5LDMzLjM3LDI2LjU5WiIvPjwvZz48L3N2Zz4=\",\"srcOrientation\":\"horizontal\"},\"position\":[0,0,1,1],\"scaleMode\":\"0\"}},{\"name\":\"ForegroundImageComponent\",\"settings\":{\"image\":{\"size\":[0,0],\"src\":\"default\",\"srcOrientation\":[]},\"isForeground\":1,\"position\":[0,0,1,1],\"scaleMode\":\"0\"}}],\"settings\":{\"BindingType\":\"param\",\"aspectRatio\":3.7777777777777777,\"backgroundColor\":[0,0,0,\"1\"],\"backgroundOffset\":0,\"backgroundOpacity\":1,\"fixedAspectRatio\":\"off\",\"foregroundColor\":[252,252,196],\"orientation\":\"vertical\",\"showBackgroundColor\":false,\"value\":0,\"version\":\"R2022b\"},\"type\":\"LinearGauge\"}"
  X140 : ToggleSwitchBlock  LabelPosition=Bottom
      settings: Values={{'Off', 'On'}, [0 1]}

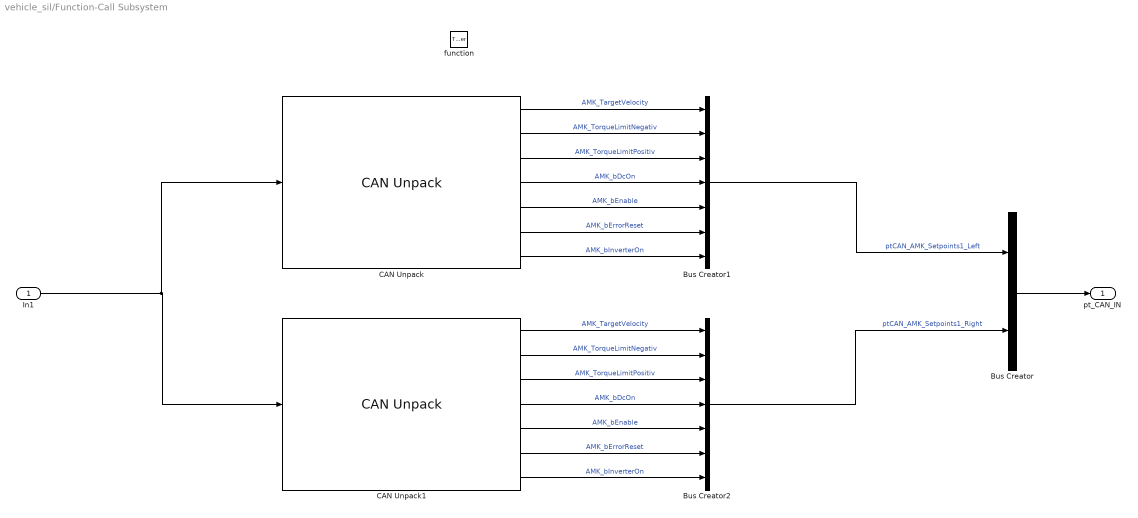
== system vehicle_sil/Function-Call Subsystem ==
  In1 : Inport
  function : TriggerPort  TriggerType=function-call  VariantControl=(inherit)
  Bus Creator : BusCreator  Inputs=2
  Bus Creator1 : BusCreator  Inputs=7
  Bus Creator2 : BusCreator  Inputs=7
  CAN Unpack : canmsglib/CAN Unpack  CANdbFile=C:\Users\LinF\Documents\MACFE\Embedded\CAN_Stuff\CAN_Databases\CAN_AMKInverter.dbc  MsgList=AMK0_SetPoints1  MsgName=AMK0_SetPoints1  MsgIDType=Standard (11-bit identifier)  MsgIdentifier=389  MsgLength=8  SignalInfo={'AMK_TargetVelocity','16','16','LE','signed','Standard','0','1','0','-Inf','Inf';'AMK_TorqueLimitNegativ','48','16','LE','signed','Standard','0','1','0','-Inf','Inf';'AMK_TorqueLimitPositiv','32','16','LE','signed','Standard','0','1','0','-Inf','Inf';'AMK_bDcOn','9','1','LE','unsigned','Standard','0','1','0','-Inf','Inf';'AMK_bEnable','10','1','LE','unsigned','Standard','0','1','0','-Inf','Inf';'AMK_bErrorReset','11','1','LE','unsigned','Standard','0','1','0','-Inf','Inf';'AMK_bInverterOn','8','1','LE','unsigned','Standard','0','1','0','-Inf','Inf'}  IDPort=off  TimestampPort=off  ErrorPort=off  RemotePort=off  LengthPort=off  StatusPort=off  ApplyMinMax=off
      settings: LibrarySourceBlock=canlib/CAN Unpack  DataFormat=CANdb specified signals
  CAN Unpack1 : canmsglib/CAN Unpack  CANdbFile=C:\Users\LinF\Documents\MACFE\Embedded\CAN_Stuff\CAN_Databases\CAN_AMKInverter.dbc  MsgList=AMK1_SetPoints1  MsgName=AMK1_SetPoints1  MsgIDType=Standard (11-bit identifier)  MsgIdentifier=390  MsgLength=8  SignalInfo={'AMK_TargetVelocity','16','16','LE','signed','Standard','0','1','0','-Inf','Inf';'AMK_TorqueLimitNegativ','48','16','LE','signed','Standard','0','1','0','-Inf','Inf';'AMK_TorqueLimitPositiv','32','16','LE','signed','Standard','0','1','0','-Inf','Inf';'AMK_bDcOn','9','1','LE','unsigned','Standard','0','1','0','-Inf','Inf';'AMK_bEnable','10','1','LE','unsigned','Standard','0','1','0','-Inf','Inf';'AMK_bErrorReset','11','1','LE','unsigned','Standard','0','1','0','-Inf','Inf';'AMK_bInverterOn','8','1','LE','unsigned','Standard','0','1','0','-Inf','Inf'}  IDPort=off  TimestampPort=off  ErrorPort=off  RemotePort=off  LengthPort=off  StatusPort=off  ApplyMinMax=off
      settings: LibrarySourceBlock=canlib/CAN Unpack  DataFormat=CANdb specified signals
  pt_CAN_IN : Outport
  wires:
  Bus Creator/1 -> pt_CAN_IN/1
  Bus Creator2/1 -> Bus Creator/2  "ptCAN_AMK_Setpoints1_Right"
  Bus Creator1/1 -> Bus Creator/1  "ptCAN_AMK_Setpoints1_Left"
  In1/1 -> CAN Unpack/1, CAN Unpack1/1
  CAN Unpack/1 -> Bus Creator1/1  "AMK_TargetVelocity"
  CAN Unpack/2 -> Bus Creator1/2  "AMK_TorqueLimitNegativ"
  CAN Unpack/3 -> Bus Creator1/3  "AMK_TorqueLimitPositiv"
  CAN Unpack/4 -> Bus Creator1/4  "AMK_bDcOn"
  CAN Unpack/5 -> Bus Creator1/5  "AMK_bEnable"
  CAN Unpack/6 -> Bus Creator1/6  "AMK_bErrorReset"
  CAN Unpack/7 -> Bus Creator1/7  "AMK_bInverterOn"
  CAN Unpack1/3 -> Bus Creator2/3  "AMK_TorqueLimitPositiv"
  CAN Unpack1/6 -> Bus Creator2/6  "AMK_bErrorReset"
  CAN Unpack1/4 -> Bus Creator2/4  "AMK_bDcOn"
  CAN Unpack1/7 -> Bus Creator2/7  "AMK_bInverterOn"
  CAN Unpack1/2 -> Bus Creator2/2  "AMK_TorqueLimitNegativ"
  CAN Unpack1/5 -> Bus Creator2/5  "AMK_bEnable"
  CAN Unpack1/1 -> Bus Creator2/1  "AMK_TargetVelocity"

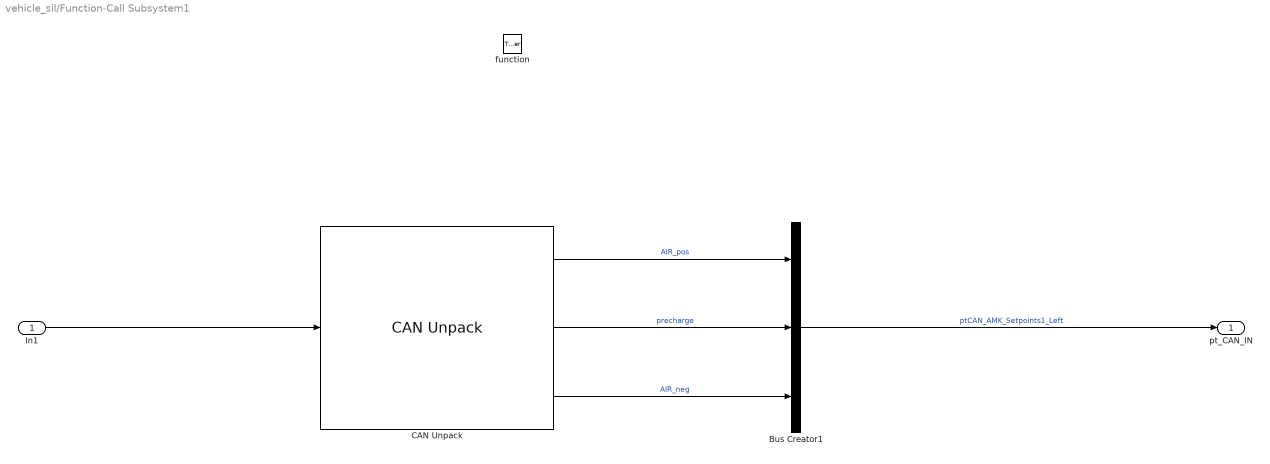
== system vehicle_sil/Function-Call Subsystem1 ==
  In1 : Inport
  function : TriggerPort  TriggerType=function-call  VariantControl=(inherit)
  Bus Creator1 : BusCreator  Inputs=3
  CAN Unpack : canmsglib/CAN Unpack  CANdbFile=C:\Users\LinF\Documents\MACFE\Embedded\CAN_Databases\BMS.dbc  MsgList=MSGID_0X622  MsgName=MSGID_0X622  MsgIDType=Standard (11-bit identifier)  MsgIdentifier=1570  MsgLength=3  SignalInfo={'MPO2_State','16','8','BE','unsigned','Standard','0','1','0','-Inf','Inf';'MPO4_State','8','8','BE','unsigned','Standard','0','1','0','-Inf','Inf';'MPO_State','0','8','BE','unsigned','Standard','0','1','0','-Inf','Inf'}  IDPort=off  TimestampPort=off  ErrorPort=off  RemotePort=off  LengthPort=off  StatusPort=off  ApplyMinMax=off
      settings: LibrarySourceBlock=canlib/CAN Unpack  DataFormat=CANdb specified signals
  pt_CAN_IN : Outport
  wires:
  Bus Creator1/1 -> pt_CAN_IN/1  "ptCAN_AMK_Setpoints1_Left"
  In1/1 -> CAN Unpack/1
  CAN Unpack/3 -> Bus Creator1/3  "AIR_neg"
  CAN Unpack/1 -> Bus Creator1/1  "AIR_pos"
  CAN Unpack/2 -> Bus Creator1/2  "precharge"

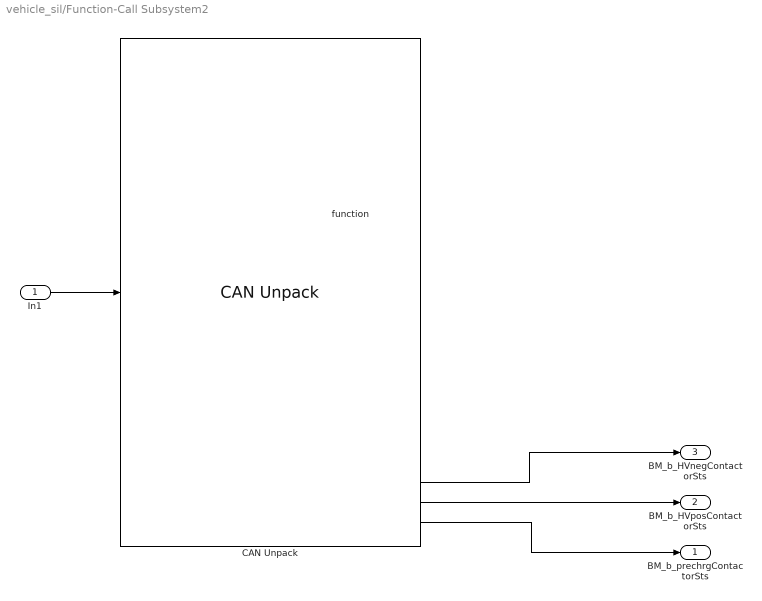
== system vehicle_sil/Function-Call Subsystem2 ==
  In1 : Inport
  function : TriggerPort  TriggerType=function-call  VariantControl=(inherit)
  CAN Unpack : canmsglib/CAN Unpack  CANdbFile=C:\Users\LinF\Documents\MACFE\Embedded\CAN_Databases\BMS.dbc  MsgList=MSGID_0X626  MsgName=MSGID_0X626  MsgIDType=Standard (11-bit identifier)  MsgIdentifier=1574  MsgLength=3  SignalInfo={'Blank','1','1','LE','unsigned','Standard','0','1','0','0','1';'Blank','2','1','LE','unsigned','Standard','0','1','0','0','1';'Blank','3','1','LE','unsigned','Standard','0','1','0','0','1';'Blank','4','1','LE','unsigned','Standard','0','1','0','0','1';'Blank','5','1','LE','unsigned','Standard','0','1','0','0','1';'Blank','6','1','LE','unsigned','Standard','0','1','0','0','1';'Blank','7','1','LE','unsigned','Standard','0','1','0','0','1';'Blank','9','1','LE','unsigned','Standard','0','1','0','0','1';'Blank','10','1','LE','unsigned','Standard','0','1','0','0','1';'Blank','11','1','LE','unsigned','Standard','0','1','0','0','1';'Blank','12','1','LE','unsigned','Standard','0','1','0','0','1';'Blank','13','1','LE','unsigned','Standard','0','1','0','0','1';'Blank','14','1','LE','unsigned','Standard','0','1','0','0','1';'Blank','15','1','LE','unsigned','Standard','0','1','0','0','1';'Blank','17','1','LE','unsigned','Standard','0','1','0','0','1';'Blank','18','1','LE','unsigned','Standard','0','1','0','0','1';'Blank','19','1','LE','unsigned','Standard','0','1','0','0','1';'Blank','20','1','LE','unsigned','Standard','0','1','0','0','1';'Blank','21','1','LE','unsigned','Standard','0','1','0','0','1';'Blank','22','1','LE','unsigned','Standard','0','1','0','0','1';'Blank','23','1','LE','unsigned','Standard','0','1','0','0','1';'MultiPurpose_Output','0','1','LE','unsigned','Standard','0','1','0','0','1';'MultiPurpose_Output_2','8','1','LE','unsigned','Standard','0','1','0','0','1';'MultiPurpose_Output_4','16','1','LE','unsigned','Standard','0','1','0','0','1'}  IDPort=off  TimestampPort=off  ErrorPort=off  RemotePort=off  LengthPort=off  StatusPort=off  ApplyMinMax=off
      settings: LibrarySourceBlock=canlib/CAN Unpack  DataFormat=CANdb specified signals
  BM_b_prechrgContactorSts : Outport
  BM_b_HVposContactorSts : Outport  Port=2
  BM_b_HVnegContactorSts : Outport  Port=3
  wires:
  In1/1 -> CAN Unpack/1
  CAN Unpack/24 -> BM_b_prechrgContactorSts/1
  CAN Unpack/22 -> BM_b_HVnegContactorSts/1
  CAN Unpack/23 -> BM_b_HVposContactorSts/1

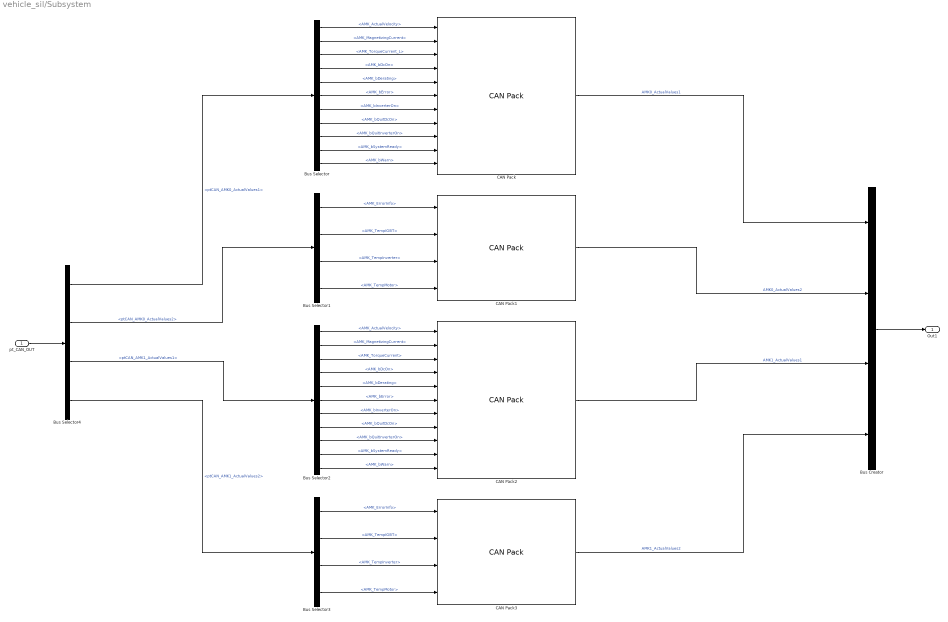
== system vehicle_sil/Subsystem ==
  pt_CAN_OUT : Inport
  Bus Creator : BusCreator  Inputs=4
  Bus Selector : BusSelector  OutputSignals=AMK_ActualVelocity,AMK_MagnetizingCurrent,AMK_TorqueCurrent_L,AMK_bDcOn,AMK_bDerating,AMK_bError,AMK_bInverterOn,AMK_bQuitDcOn,AMK_bQuitInverterOn,AMK_bSystemReady,AMK_bWarn
  Bus Selector1 : BusSelector  OutputSignals=AMK_ErrorInfo,AMK_TempIGBT,AMK_TempInverter,AMK_TempMotor
  Bus Selector2 : BusSelector  OutputSignals=AMK_ActualVelocity,AMK_MagnetizingCurrent,AMK_TorqueCurrent,AMK_bDcOn,AMK_bDerating,AMK_bError,AMK_bInverterOn,AMK_bQuitDcOn,AMK_bQuitInverterOn,AMK_bSystemReady,AMK_bWarn
  Bus Selector3 : BusSelector  OutputSignals=AMK_ErrorInfo,AMK_TempIGBT,AMK_TempInverter,AMK_TempMotor
  Bus Selector4 : BusSelector  OutputSignals=ptCAN_AMK0_ActualValues1,ptCAN_AMK0_ActualValues2,ptCAN_AMK1_ActualValues1,ptCAN_AMK1_ActualValues2
  CAN Pack : canmsglib/CAN Pack  CANdbFile=C:\Users\LinF\Documents\MACFE\Embedded\CAN_Stuff\CAN_Databases\CAN_AMKInverter.dbc  MsgList=AMK0_ActualValues1  MsgName=AMK0_ActualValues1  MsgIDType=Standard (11-bit identifier)  MsgIdentifier=644  MsgLength=8  Remote=off  ApplyMinMax=off  BusOutput=off  SignalInfo={'AMK_ActualVelocity','16','16','LE','signed','Standard','0','1','0','-Inf','Inf';'AMK_MagnetizingCurrent','48','16','LE','signed','Standard','0','1','0','-Inf','Inf';'AMK_TorqueCurrent','32','16','LE','signed','Standard','0','1','0','-Inf','Inf';'AMK_bDcOn','12','1','LE','unsigned','Standard','0','1','0','-Inf','Inf';'AMK_bDerating','15','1','LE','unsigned','Standard','0','1','0','-Inf','Inf';'AMK_bError','9','1','LE','unsigned','Standard','0','1','0','-Inf','Inf';'AMK_bInverterOn','14','1','LE','unsigned','Standard','0','1','0','-Inf','Inf';'AMK_bQuitDcOn','11','1','LE','unsigned','Standard','0','1','0','-Inf','Inf';'AMK_bQuitInverterOn','13','1','LE','unsigned','Standard','0','1','0','-Inf','Inf';'AMK_bSystemReady','8','1','LE','unsigned','Standard','0','1','0','-Inf','Inf';'AMK_bWarn','10','1','LE','unsigned','Standard','0','1','0','-Inf','Inf'}
      settings: LibrarySourceBlock=canlib/CAN Pack  DataFormat=CANdb specified signals
  CAN Pack1 : canmsglib/CAN Pack  CANdbFile=C:\Users\LinF\Documents\MACFE\Embedded\CAN_Stuff\CAN_Databases\CAN_AMKInverter.dbc  MsgList=AMK0_ActualValues2  MsgName=AMK0_ActualValues2  MsgIDType=Standard (11-bit identifier)  MsgIdentifier=646  MsgLength=8  Remote=off  ApplyMinMax=off  BusOutput=off  SignalInfo={'AMK_ErrorInfo','32','16','LE','unsigned','Standard','0','1','0','0','65535';'AMK_TempIGBT','48','16','LE','signed','Standard','0','0.1','0','-3276.8','3276.7';'AMK_TempInverter','16','16','LE','signed','Standard','0','0.1','0','-3276.8','3276.7';'AMK_TempMotor','0','16','LE','signed','Standard','0','0.1','0','-3276.8','3276.7'}
      settings: LibrarySourceBlock=canlib/CAN Pack  DataFormat=CANdb specified signals
  CAN Pack2 : canmsglib/CAN Pack  CANdbFile=C:\Users\LinF\Documents\MACFE\Embedded\CAN_Stuff\CAN_Databases\CAN_AMKInverter.dbc  MsgList=AMK1_ActualValues1  MsgName=AMK1_ActualValues1  MsgIDType=Standard (11-bit identifier)  MsgIdentifier=645  MsgLength=8  Remote=off  ApplyMinMax=off  BusOutput=off  SignalInfo={'AMK_ActualVelocity','16','16','LE','signed','Standard','0','1','0','-Inf','Inf';'AMK_MagnetizingCurrent','48','16','LE','signed','Standard','0','1','0','-Inf','Inf';'AMK_TorqueCurrent','32','16','LE','signed','Standard','0','1','0','-Inf','Inf';'AMK_bDcOn','12','1','LE','unsigned','Standard','0','1','0','-Inf','Inf';'AMK_bDerating','15','1','LE','unsigned','Standard','0','1','0','-Inf','Inf';'AMK_bError','9','1','LE','unsigned','Standard','0','1','0','-Inf','Inf';'AMK_bInverterOn','14','1','LE','unsigned','Standard','0','1','0','-Inf','Inf';'AMK_bQuitDcOn','11','1','LE','unsigned','Standard','0','1','0','-Inf','Inf';'AMK_bQuitInverterOn','13','1','LE','unsigned','Standard','0','1','0','-Inf','Inf';'AMK_bSystemReady','8','1','LE','unsigned','Standard','0','1','0','-Inf','Inf';'AMK_bWarn','10','1','LE','unsigned','Standard','0','1','0','-Inf','Inf'}
      settings: LibrarySourceBlock=canlib/CAN Pack  DataFormat=CANdb specified signals
  CAN Pack3 : canmsglib/CAN Pack  CANdbFile=C:\Users\LinF\Documents\MACFE\Embedded\CAN_Stuff\CAN_Databases\CAN_AMKInverter.dbc  MsgList=AMK1_ActualValues2  MsgName=AMK1_ActualValues2  MsgIDType=Standard (11-bit identifier)  MsgIdentifier=647  MsgLength=8  Remote=off  ApplyMinMax=off  BusOutput=off  SignalInfo={'AMK_ErrorInfo','32','16','LE','unsigned','Standard','0','1','0','0','65535';'AMK_TempIGBT','48','16','LE','signed','Standard','0','0.1','0','-3276.8','3276.7';'AMK_TempInverter','16','16','LE','signed','Standard','0','0.1','0','-3276.8','3276.7';'AMK_TempMotor','0','16','LE','signed','Standard','0','0.1','0','-3276.8','3276.7'}
      settings: LibrarySourceBlock=canlib/CAN Pack  DataFormat=CANdb specified signals
  Out1 : Outport
  wires:
  CAN Pack/1 -> Bus Creator/1  "AMK0_ActualValues1"
  CAN Pack1/1 -> Bus Creator/2  "AMK0_ActualValues2"
  CAN Pack2/1 -> Bus Creator/3  "AMK1_ActualValues1"
  CAN Pack3/1 -> Bus Creator/4  "AMK1_ActualValues2"
  Bus Selector4/1 -> Bus Selector/1  "<ptCAN_AMK0_ActualValues1>"
  Bus Selector4/2 -> Bus Selector1/1  "<ptCAN_AMK0_ActualValues2>"
  Bus Selector4/3 -> Bus Selector2/1  "<ptCAN_AMK1_ActualValues1>"
  Bus Selector4/4 -> Bus Selector3/1  "<ptCAN_AMK1_ActualValues2>"
  pt_CAN_OUT/1 -> Bus Selector4/1
  Bus Creator/1 -> Out1/1
  Bus Selector/1 -> CAN Pack/1  "<AMK_ActualVelocity>"
  Bus Selector/3 -> CAN Pack/3  "<AMK_TorqueCurrent_L>"
  Bus Selector/2 -> CAN Pack/2  "<AMK_MagnetizingCurrent>"
  Bus Selector/4 -> CAN Pack/4  "<AMK_bDcOn>"
  Bus Selector/5 -> CAN Pack/5  "<AMK_bDerating>"
  Bus Selector/6 -> CAN Pack/6  "<AMK_bError>"
  Bus Selector/7 -> CAN Pack/7  "<AMK_bInverterOn>"
  Bus Selector/8 -> CAN Pack/8  "<AMK_bQuitDcOn>"
  Bus Selector/9 -> CAN Pack/9  "<AMK_bQuitInverterOn>"
  Bus Selector/10 -> CAN Pack/10  "<AMK_bSystemReady>"
  Bus Selector/11 -> CAN Pack/11  "<AMK_bWarn>"
  Bus Selector1/1 -> CAN Pack1/1  "<AMK_ErrorInfo>"
  Bus Selector1/2 -> CAN Pack1/2  "<AMK_TempIGBT>"
  Bus Selector1/3 -> CAN Pack1/3  "<AMK_TempInverter>"
  Bus Selector1/4 -> CAN Pack1/4  "<AMK_TempMotor>"
  Bus Selector2/3 -> CAN Pack2/3  "<AMK_TorqueCurrent>"
  Bus Selector3/1 -> CAN Pack3/1  "<AMK_ErrorInfo>"
  Bus Selector2/7 -> CAN Pack2/7  "<AMK_bInverterOn>"
  Bus Selector2/4 -> CAN Pack2/4  "<AMK_bDcOn>"
  Bus Selector2/2 -> CAN Pack2/2  "<AMK_MagnetizingCurrent>"
  Bus Selector3/4 -> CAN Pack3/4  "<AMK_TempMotor>"
  Bus Selector3/2 -> CAN Pack3/2  "<AMK_TempIGBT>"
  Bus Selector2/5 -> CAN Pack2/5  "<AMK_bDerating>"
  Bus Selector2/10 -> CAN Pack2/10  "<AMK_bSystemReady>"
  Bus Selector3/3 -> CAN Pack3/3  "<AMK_TempInverter>"
  Bus Selector2/8 -> CAN Pack2/8  "<AMK_bQuitDcOn>"
  Bus Selector2/6 -> CAN Pack2/6  "<AMK_bError>"
  Bus Selector2/11 -> CAN Pack2/11  "<AMK_bWarn>"
  Bus Selector2/1 -> CAN Pack2/1  "<AMK_ActualVelocity>"
  Bus Selector2/9 -> CAN Pack2/9  "<AMK_bQuitInverterOn>"

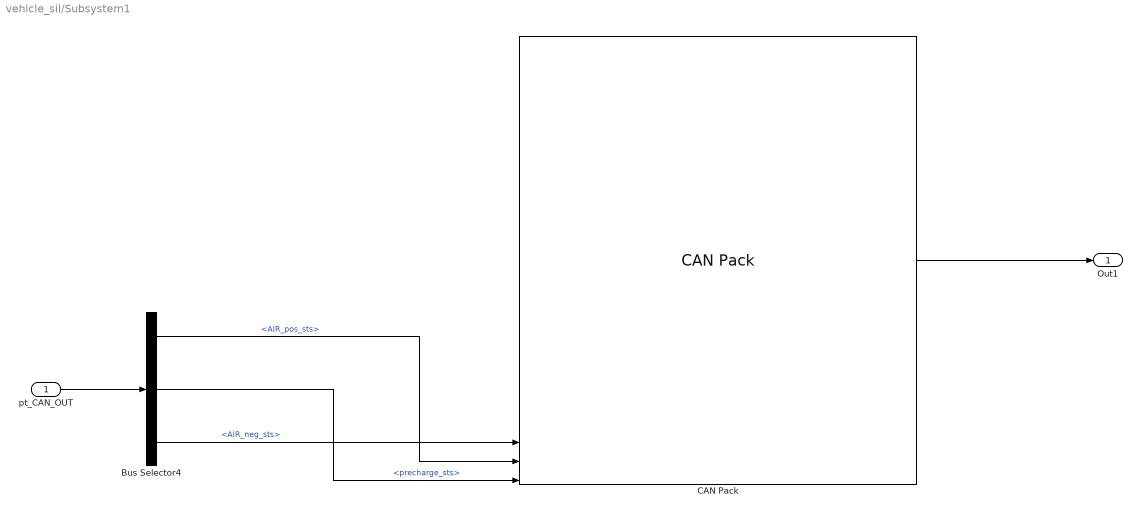
== system vehicle_sil/Subsystem1 ==
  pt_CAN_OUT : Inport
  Bus Selector4 : BusSelector  OutputSignals=AIR_pos_sts,precharge_sts,AIR_neg_sts
  CAN Pack : canmsglib/CAN Pack  CANdbFile=C:\Users\LinF\Documents\MACFE\Embedded\CAN_Databases\BMS.dbc  MsgList=MSGID_0X626  MsgName=MSGID_0X626  MsgIDType=Standard (11-bit identifier)  MsgIdentifier=1574  MsgLength=3  Remote=off  ApplyMinMax=off  BusOutput=off  SignalInfo={'Blank','1','1','LE','unsigned','Standard','0','1','0','0','1';'Blank','2','1','LE','unsigned','Standard','0','1','0','0','1';'Blank','3','1','LE','unsigned','Standard','0','1','0','0','1';'Blank','4','1','LE','unsigned','Standard','0','1','0','0','1';'Blank','5','1','LE','unsigned','Standard','0','1','0','0','1';'Blank','6','1','LE','unsigned','Standard','0','1','0','0','1';'Blank','7','1','LE','unsigned','Standard','0','1','0','0','1';'Blank','9','1','LE','unsigned','Standard','0','1','0','0','1';'Blank','10','1','LE','unsigned','Standard','0','1','0','0','1';'Blank','11','1','LE','unsigned','Standard','0','1','0','0','1';'Blank','12','1','LE','unsigned','Standard','0','1','0','0','1';'Blank','13','1','LE','unsigned','Standard','0','1','0','0','1';'Blank','14','1','LE','unsigned','Standard','0','1','0','0','1';'Blank','15','1','LE','unsigned','Standard','0','1','0','0','1';'Blank','17','1','LE','unsigned','Standard','0','1','0','0','1';'Blank','18','1','LE','unsigned','Standard','0','1','0','0','1';'Blank','19','1','LE','unsigned','Standard','0','1','0','0','1';'Blank','20','1','LE','unsigned','Standard','0','1','0','0','1';'Blank','21','1','LE','unsigned','Standard','0','1','0','0','1';'Blank','22','1','LE','unsigned','Standard','0','1','0','0','1';'Blank','23','1','LE','unsigned','Standard','0','1','0','0','1';'MultiPurpose_Output','0','1','LE','unsigned','Standard','0','1','0','0','1';'MultiPurpose_Output_2','8','1','LE','unsigned','Standard','0','1','0','0','1';'MultiPurpose_Output_4','16','1','LE','unsigned','Standard','0','1','0','0','1'}
      settings: LibrarySourceBlock=canlib/CAN Pack  DataFormat=CANdb specified signals
  Out1 : Outport
  wires:
  pt_CAN_OUT/1 -> Bus Selector4/1
  Bus Selector4/1 -> CAN Pack/23  "<AIR_pos_sts>"
  Bus Selector4/2 -> CAN Pack/24  "<precharge_sts>"
  Bus Selector4/3 -> CAN Pack/22  "<AIR_neg_sts>"
  CAN Pack/1 -> Out1/1
